simulink model "ecm_1rc"  (R2025b)
settings: Solver=VariableStepAuto  StartTime=0.0  StopTime=3347  RelTol=1e-3
undefined symbols (not defined in the file): OCV_table, SOC_brkpts
settings Model: Creator=Krupal Babariya  LastModifiedBy=Krupal Babariya

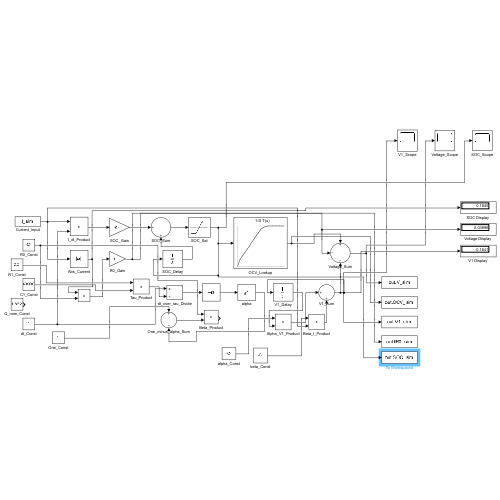
[thumbnail: Simulink's stored preview of the top-level diagram]
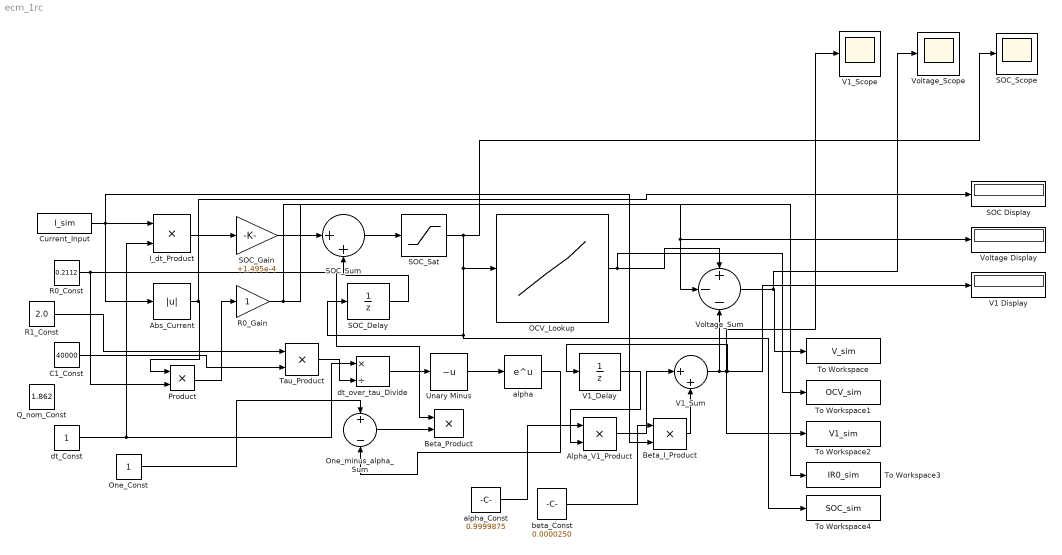
== system ecm_1rc ==
  Abs_Current : Abs  SaturateOnIntegerOverflow=off
  Alpha_V1_Product : Product
  Beta_I_Product : Product
  Beta_Product : Product
  C1_Const : Constant  Value=40000
  Current_Input : FromWorkspace  VariableName=I_sim  OutDataTypeStr=double  SampleTime=1
  I_dt_Product : Product
  OCV_Lookup : Lookup_n-D  NumberOfTableDimensions=1  BreakpointsForDimension1=SOC_brkpts  Table=OCV_table  ExtrapMethod=Clip  InternalRulePriority=Speed  RndMeth=Simplest
  One_Const : Constant
  One_minus_alpha_Sum : Sum  Inputs=+-
  Product : Product
  Q_nom_Const : Constant  Value=1.862
  R0_Const : Constant  Value=0.2112
  R0_Gain : Gain
  R1_Const : Constant  Value=2.0
  "SOC Display " : Display
  SOC_Delay : UnitDelay  InitialCondition=1  SampleTime=-1  HasFrameUpgradeWarning=on
  SOC_Gain : Gain  Gain=+1.495e-4
  SOC_Sat : Saturate  UpperLimit=1  LowerLimit=0
  SOC_Scope : Scope
      settings: ActiveDisplayYMinimum=0.735830231433191  ActiveDisplayYMaximum=1.1318165513210707
  SOC_Sum : Sum  Inputs=|++
  Tau_Product : Product
  To Workspace : ToWorkspace  VariableName=V_sim  SampleTime=-1
  To Workspace1 : ToWorkspace  VariableName=OCV_sim  SampleTime=-1
  To Workspace2 : ToWorkspace  VariableName=V1_sim  SampleTime=-1
  To Workspace3 : ToWorkspace  VariableName=IR0_sim  SampleTime=-1
  To Workspace4 : ToWorkspace  VariableName=SOC_sim  SampleTime=-1
  Unary Minus : UnaryMinus
  "V1 Display " : Display
  V1_Delay : UnitDelay  HasFrameUpgradeWarning=on
  V1_Scope : Scope
      settings: ActiveDisplayYMinimum=-0.063554536401721026  ActiveDisplayYMaximum=0.070455027660779032  DataLoggingVariableName=ScopeData2
  V1_Sum : Sum  Inputs=|++
  "Voltage Display " : Display
  Voltage_Scope : Scope
      settings: ActiveDisplayYMinimum=2.9099758653209111  ActiveDisplayYMaximum=4.9727923513418464
  Voltage_Sum : Sum  Inputs=+--
  alpha : Math
  alpha_Const : Constant  Value=0.9999875
  beta_Const : Constant  Value=0.0000250
  dt_Const : Constant
  dt_over_tau_Divide : Product  Inputs=*/
  wires:
  Current_Input/1 -> Beta_I_Product/2, Abs_Current/1, I_dt_Product/1
  dt_Const/1 -> dt_over_tau_Divide/1, I_dt_Product/2
  I_dt_Product/1 -> SOC_Gain/1
  SOC_Gain/1 -> SOC_Sum/1
  SOC_Delay/1 -> SOC_Sum/2
  SOC_Sum/1 -> SOC_Sat/1
  SOC_Sat/1 -> SOC_Scope/1, OCV_Lookup/1, To Workspace4/1, SOC_Delay/1
  R1_Const/1 -> Tau_Product/1
  C1_Const/1 -> Tau_Product/2
  Tau_Product/1 -> dt_over_tau_Divide/2
  dt_over_tau_Divide/1 -> Unary Minus/1
  Unary Minus/1 -> alpha/1
  One_Const/1 -> One_minus_alpha_Sum/1
  alpha/1 -> One_minus_alpha_Sum/2
  R0_Const/1 -> Product/2, Beta_Product/1
  One_minus_alpha_Sum/1 -> Beta_Product/2
  V1_Delay/1 -> Alpha_V1_Product/2
  Alpha_V1_Product/1 -> V1_Sum/1
  Beta_I_Product/1 -> V1_Sum/2
  V1_Sum/1 -> Voltage_Sum/3, "V1 Display "/1, V1_Delay/1, To Workspace2/1, V1_Scope/1
  OCV_Lookup/1 -> To Workspace1/1, Voltage_Sum/1
  R0_Gain/1 -> To Workspace3/1, Voltage_Sum/2, "Voltage Display "/1
  Voltage_Sum/1 -> Voltage_Scope/1, To Workspace/1
  Abs_Current/1 -> "SOC Display "/1, Product/1
  Product/1 -> R0_Gain/1
  alpha_Const/1 -> Alpha_V1_Product/1
  beta_Const/1 -> Beta_I_Product/1
